simulink model "simpowersystems_simple_phasor"  (Simulink 7.7)
settings: Solver=ode45  StartTime=0.0  StopTime=5  MaxStep=1/60  RelTol=1e-3
libraries: powerlib x5
settings Model: Creator=sfrank1  LastModifiedBy=sfrank1

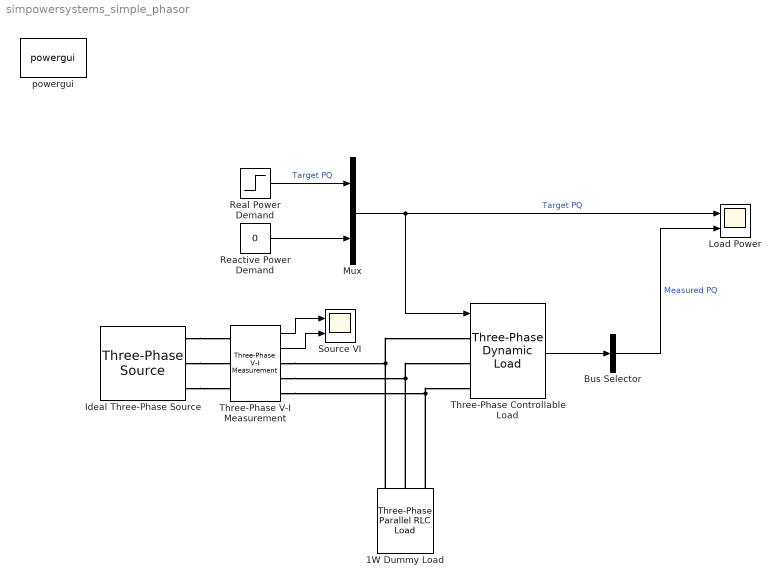
== system simpowersystems_simple_phasor ==
  1W Dummy Load : powerlib/Elements/Three-Phase Parallel RLC Load  PhysicalDomain=powersysdomain  SubClassName=unknown  LeftPortType=p1  RightPortType=p1  LConnTagsString=A|B|C  Configuration=Y (grounded)  NominalVoltage=480  NominalFrequency=60  ActivePower=1  InductivePower=0  CapacitivePower=0  Measurements=None  LoadType=constant Z
  Bus Selector : BusSelector  OutputSignals=Active power P (W),Reactive power Q (var)  OutputAsBus=on
  Ideal Three-Phase Source : powerlib/Electrical Sources/Three-Phase Source  SystemSampleTime=-1  Voltage=480  PhaseAngle=0  Frequency=60  InternalConnection=Yg  SpecifyImpedance=on  Resistance=0  Inductance=0  ShortCircuitLevel=100e3  BaseVoltage=480  XRratio=1  BusType=swing  Pref=0  Qref=0  Qmin=-inf  Qmax=inf
  Load Power : Scope  NumInputPorts=2
      settings: TickLabels=on  YMin=-5~-5  YMax=5~5
  Mux : Mux  Inputs=2
  Reactive Power Demand : Constant  Value=0
  Real Power Demand : Step  Time=2  Before=5e3  After=10e3  SampleTime=0
  Source VI : Scope  NumInputPorts=2
      settings: TickLabels=on  YMin=-5~-5  YMax=5~5
  Three-Phase Controllable Load : powerlib/Elements/Three-Phase Dynamic Load  SystemSampleTime=-1  NominalVoltage=[480 60]  ActiveReactivePowers=[100e3 0e3]  PositiveSequence=[1 0]  ExternalControl=on  NpNq=[0 0]  TimeConstants="[0  0  0  0]"  MinimumVoltage=0.7  LoadFlowParameters=[4,0,0,0,0]
  Three-Phase V-I Measurement : powerlib/Measurements/Three-Phase V-I Measurement  SystemSampleTime=-1  VoltageMeasurement=phase-to-ground  SetLabelV=off  LabelV=Vabc  Vpu=off  VpuLL=off  CurrentMeasurement=yes  SetLabelI=off  LabelI=Iabc  Ipu=off  Pbase=100e6  Vbase=500e3  OutputType=Magnitude  PhasorSimulation=on  PSBequivalent=0
  powergui : powerlib/powergui  Priority=1  SystemSampleTime=-1  SimulationMode=Phasor  SampleTime=50e-6  frequency=60  SPID=off  DisableSnubberDevices=off  DisableRonSwitches=off  DisableVfSwitches=off  SwTol=0  Interpol=off  DisplayEquations=off  FunctionMessages=off  frequencyindice=60  Pbase=100e3  ErrMax=1e-4  Iterations=50  UnitsV=kV  UnitsW=MW  echomessages=off  HookPort=off  EnableUseOfTLC=off  x0status=blocks  RestoreLinks=warning  ResistiveCurrentMeasurement=off  Ylog=off  Xlog=on  ShowGrid=off  save=off  variable=ZData  ZoomFFT=off  StartTime=0.0  cycles=1  DisplayStyle=1  FreqAxis=off  MaxFrequency=1000  frequencyindicesteady=1  display=off  methode=off
  wires:
  Reactive Power Demand/1 -> Mux/2
  Real Power Demand/1 -> Mux/1  "Target PQ"
  Mux/1 -> Three-Phase Controllable Load/1, Load Power/1  "Target PQ"
  Three-Phase Controllable Load/1 -> Bus Selector/1
  Bus Selector/1 -> Load Power/2  "Measured PQ"
  Three-Phase V-I Measurement/1 -> Source VI/1
  Three-Phase V-I Measurement/2 -> Source VI/2
  connections:
  1W Dummy Load/LConn1 -- Three-Phase Controllable Load/LConn1 -- Three-Phase V-I Measurement/RConn1
  1W Dummy Load/LConn2 -- Three-Phase Controllable Load/LConn2 -- Three-Phase V-I Measurement/RConn2
  1W Dummy Load/LConn3 -- Three-Phase Controllable Load/LConn3 -- Three-Phase V-I Measurement/RConn3
  Ideal Three-Phase Source/RConn1 -- Three-Phase V-I Measurement/LConn1
  Ideal Three-Phase Source/RConn2 -- Three-Phase V-I Measurement/LConn2
  Ideal Three-Phase Source/RConn3 -- Three-Phase V-I Measurement/LConn3
